simulink model "PNNFT"  (R2020b)
settings: Solver=FixedStepAuto  StartTime=0.0  StopTime=20  FixedStep=Ts  MaxStep=1e-4  RelTol=1e-4  EnableMultiTasking=on
undefined symbols (not defined in the file or in its folder): ECons, Ts
libraries: powerlib x1
settings Model: Creator=ferna  LastModifiedBy=ferna
settings DataIOCC: ReturnWorkspaceOutputs=off
settings DebuggingCC: ArithmeticOperatorsInVariantConditions=warning
settings SFSimCC: SimUseLocalCustomCode=off  CustomCodeUndefinedFunction=UseInterfaceOnly
settings RTWCC: RTWUseLocalCustomCode=off
settings CodeAppCC: StateflowObjectComments=on

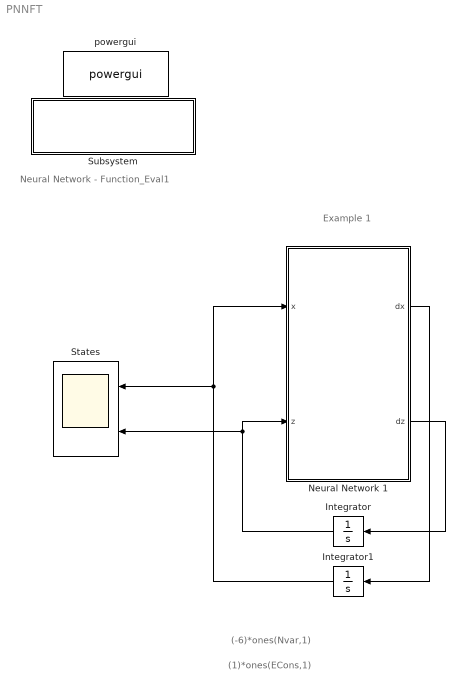
== system PNNFT ==
  note: (1)*ones(ECons,1)
  note: (-6)*ones(Nvar,1)
  note: Example 1
  note: Neural Network - Function_Eval1
  Integrator : Integrator  InitialCondition=-(6.5)*ones(ECons,1)
  Integrator1 : Integrator  InitialCondition=[-6,2.5]
  Neural Network 1 : MATLAB Function  TreatAsAtomicUnit=on
  States : Scope  NumInputPorts=2
  Subsystem : Subsystem
      settings: OpenFcn=open_system('power_new_palette')
      mask Display: disp(sprintf('Open Simscape Power Systems\n(Specialized Technology)\nPalette Library'));
  powergui : powerlib/powergui  Priority=1  SimulationMode=Continuous  SampleTime=Ts  frequency=60  Iterations=50  frequencyindice=60  Pbase=100e6  ErrMax=1e-4  UnitsV=kV  UnitsW=MW  buscounter=0  FunctionMessages=off  echomessages=off  EnableUseOfTLC=off  CurrentSourceSwitches=off  DisableSnubberDevices=off  DisableRonSwitches=off  DisableVfSwitches=off  DisplayEquations=off  AutomaticDiscreteSolvers=off  SolverType=Tustin/Backward Euler (TBE)  Interpol=off  ExternalGateDelay=off  methode=off  Ts=100  x0status=blocks  SPID=off  SwTol=0  HookPort=off  NonlinearTolerance=1e-4  nMaxIteration=100  ContinueOnMaxIteration=off  RestoreLinks=warning  ResistiveCurrentMeasurement=off  Frange=[0:2:500]  Ylog=off  Xlog=on  ShowGrid=off  save=off  variable=ZData  structure=0  ZoomFFT=off  StartTime=0.0  cycles=1  DisplayStyle=1  fundamental=60  FreqAxis=off  MaxFrequency=1000  frequencyindicesteady=1  RmsSteady=1  display=off
  wires:
  Neural Network 1/2(dz) -> Integrator/1
  Integrator/1 -> Neural Network 1/2(z), States/2
  Neural Network 1/1(dx) -> Integrator1/1
  Integrator1/1 -> States/1, Neural Network 1/1(x)

== system PNNFT/Subsystem ==

== matlab function PNNFT/Neural Network 1 ==
  data: x input; dx output; z input; dz output
function [dx,dz] = states(x,z)
%%%%%%%%%%%%%%%%%%%%%%%%%%
%% Calling The Function %%
%%%%%%%%%%%%%%%%%%%%%%%%%%
dx = zeros(length(x),1);
dz = zeros(length(z),1);

coder.extrinsic('solveSymsN1');
[dx,dz] = solveSymsN1(x,z);

end
